simulink model "mconversion11"  (Simulink 6.3)
settings: Solver=ode3  StartTime=0.0  StopTime=10.0  RelTol=1e-3
PreLoadFcn:
  | load numericVars;
settings Model: Creator=matthewe  LastModifiedBy=matthewe  ExtModeEnableOpenProtocolUploading=on  ExtModeOpenProtocolUploadingEqualLengthVectors=off  ExtModeAutoUpdateStatusClock=off  StrictBusMsg=None
settings DataIOCC: SaveFormat=StructureWithTime  OutputSaveName=yout1,yout2,yout3,yout4,yout5,yout6  SignalLoggingName=logsOut
settings OptimizationCC: InlineParams=on  InlineInvariantSignals=on
settings DebuggingCC: CheckExecutionContextPreStartOutputMsg=on  CheckExecutionContextRuntimeOutputMsg=on  SigSpecEnsureSampleTime=on  SolverPrmCheckMsg=none
settings HardwareCC: TargetUnknown=on

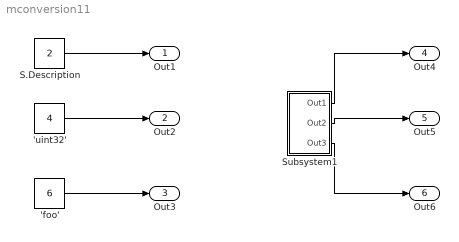
== system mconversion11 ==
  'foo' : Constant  Value=6  OutDataTypeMode=Specify via dialog  OutDataType=foo  SampleTime=0.2
  'uint32' : Constant  Value=4  OutDataTypeMode=Specify via dialog  OutDataType=S1.DataType  SampleTime=0.2
  S.Description : Constant  Value=2  OutDataTypeMode=Specify via dialog  OutDataType=S.Description  SampleTime=0.2
  Subsystem1 : Subsystem  DataTypeOverride=TrueSingles
  Out1 : Outport
  Out2 : Outport  Port=2
  Out3 : Outport  Port=3
  Out4 : Outport  Port=4
  Out5 : Outport  Port=5
  Out6 : Outport  Port=6
  wires:
  S.Description/1 -> Out1/1
  'uint32'/1 -> Out2/1
  'foo'/1 -> Out3/1
  Subsystem1/1(Out1) -> Out4/1
  Subsystem1/2(Out2) -> Out5/1
  Subsystem1/3(Out3) -> Out6/1

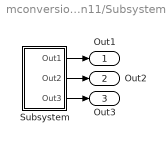
== system mconversion11/Subsystem1 ==
  Subsystem : Subsystem  TreatAsAtomicUnit=on
  Out1 : Outport
  Out2 : Outport  Port=2
  Out3 : Outport  Port=3
  wires:
  Subsystem/1(Out1) -> Out1/1
  Subsystem/2(Out2) -> Out2/1
  Subsystem/3(Out3) -> Out3/1

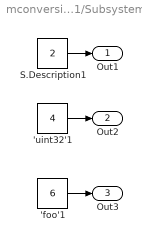
== system mconversion11/Subsystem1/Subsystem ==
  'foo'1 : Constant  Value=6  OutDataTypeMode=Specify via dialog  OutDataType=foo  SampleTime=0.2
  'uint32'1 : Constant  Value=4  OutDataTypeMode=Specify via dialog  OutDataType='uint32'  SampleTime=0.2
  S.Description1 : Constant  Value=2  OutDataTypeMode=Specify via dialog  OutDataType=S.Description  SampleTime=0.2
  Out1 : Outport
  Out2 : Outport  Port=2
  Out3 : Outport  Port=3
  wires:
  S.Description1/1 -> Out1/1
  'uint32'1/1 -> Out2/1
  'foo'1/1 -> Out3/1
